simulink model "simscape_Example_20231128_1528"  (R2023b)
settings: Solver=ode23t  StartTime=0.0  StopTime=100  RelTol=1e-3
libraries: nesl_utility x8, fl_lib x6, ee_lib x4
settings Model: Creator=Patri  LastModifiedBy=Patri

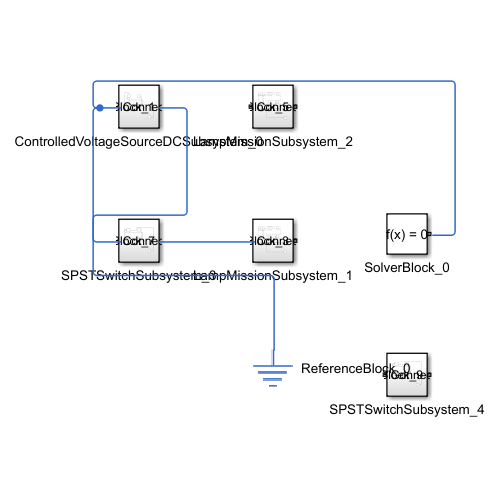
[thumbnail: Simulink's stored preview of the top-level diagram]
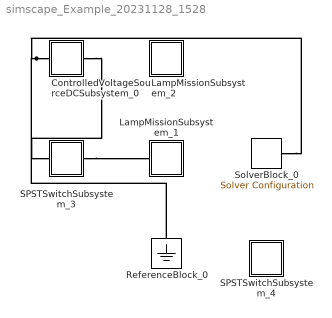
== system simscape_Example_20231128_1528 ==
  ControlledVoltageSourceDCSubsystem_0 : Subsystem
  LampMissionSubsystem_1 : Subsystem
  LampMissionSubsystem_2 : Subsystem
  ReferenceBlock_0 : fl_lib/Electrical/Electrical Elements/Electrical Reference
  SPSTSwitchSubsystem_3 : Subsystem
  SPSTSwitchSubsystem_4 : Subsystem
  SolverBlock_0 : nesl_utility/Solver Configuration  PhysicalDomain=network_engine_domain  SubClassName=solver  LeftPortType=input  RightPortType=generic  Tones=[]  Harmonics=[]  SimulateNoise=off  Profile=off  UseLocalSampling=off  EnableSwitchedLinearOptims=on  FrequencyDomain=off  UseCCode=off  RelTol=0.001  AbsTol=0.001  MinStep=1e-09  ToWorkspace=off  RevertToSquareIcSolve=off  NumHomotopyIterations=100  PhasorMode=off  PhasorModeNumHarmonics=1  ConsistencySolver=NEWTON_XTOL_AFTER_FTOL  IndexReductionMethod=DerivativeReplacement  DoDC=off  ResidualTolerance=1e-09  ConsistencyTolSource=GLOBAL  ConsistencyAbsTol=0.001  ConsistencyRelTol=0.001  ConsistencyTolFactor=0.001  UseLocalSolver=off  LocalSolverChoice=NE_BACKWARD_EULER_ADVANCER  ResolveIndetEquations=on  FunctionEvalNumThread=1  LocalSolverSampleTime=0.001  DoFixedCost=off  MaxNonlinIter=3  MaxModeIter=2  ComputeImpulses=off  ImpulseIterations=2  LinearAlgebra=auto  LinearAlgebraNumThread=0  EquationFormulation=NE_TIME_EF  DelaysMemoryBudget=1024  AutomaticFiltering=on  FilteringTimeConstant=0.001  PartitionStorageMethod=AS_NEEDED  PartitionMemoryBudget=1024  PartitionMethod=ROBUST  MultibodyUseLocalSolver=off  MultibodyLocalSolverChoice=ODE1  MultibodyLocalSolverSampleTime=0.001
  connections:
  ControlledVoltageSourceDCSubsystem_0/RConn1 -- SPSTSwitchSubsystem_3/LConn1
  SPSTSwitchSubsystem_3/RConn1 -- LampMissionSubsystem_1/LConn1
  ControlledVoltageSourceDCSubsystem_0/LConn1 -- SolverBlock_0/RConn1 -- ReferenceBlock_0/LConn1

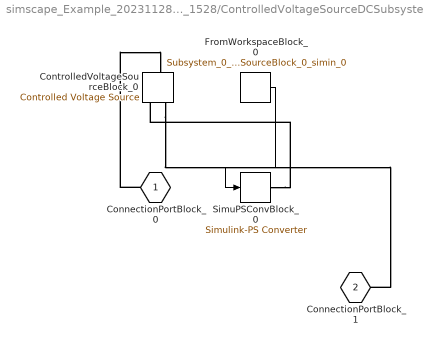
== system simscape_Example_20231128_1528/ControlledVoltageSourceDCSubsystem_0 ==
  ControlledVoltageSourceBlock_0 : fl_lib/Electrical/Electrical Sources/Controlled Voltage Source
  FromWorkspaceBlock_0 : FromWorkspace  VariableName=Subsystem_0_ControlledVoltageSourceBlock_0_simin_0
  SimuPSConvBlock_0 : nesl_utility/Simulink-PS Converter  PhysicalDomain=network_engine_domain  SubClassName=ps_input  LeftPortType=input  RightPortType=output  PseudoPeriodic=off  Frequencies=[]  NoiseDistribution=none  NoiseParameters=[]  Unit=1  AffineConversion=off  FilteringAndDerivatives=filter  SimscapeFilterOrder=1  InputFilterTimeConstant=0.001  UdotUserProvided=0
  ConnectionPortBlock_0 : PMIOPort  Side=Left
  ConnectionPortBlock_1 : PMIOPort  Port=2  Side=Right
  wires:
  FromWorkspaceBlock_0/1 -> SimuPSConvBlock_0/1
  connections:
  SimuPSConvBlock_0/RConn1 -- ControlledVoltageSourceBlock_0/RConn1
  ConnectionPortBlock_0/RConn1 -- ControlledVoltageSourceBlock_0/LConn1
  ControlledVoltageSourceBlock_0/RConn2 -- ConnectionPortBlock_1/RConn1

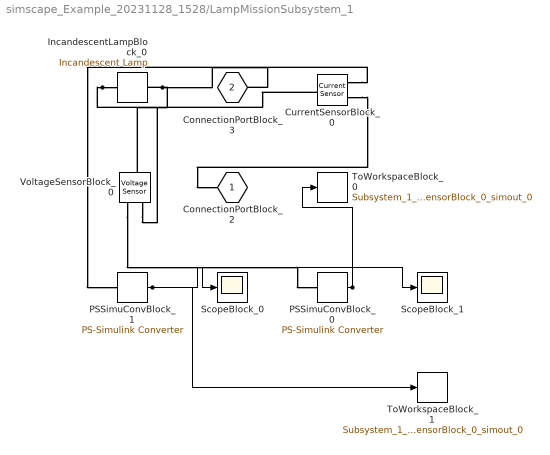
== system simscape_Example_20231128_1528/LampMissionSubsystem_1 ==
  CurrentSensorBlock_0 : fl_lib/Electrical/Electrical Sensors/Current Sensor
  IncandescentLampBlock_0 : ee_lib/Passive/Incandescent Lamp  R_param=ee.enum.passive.lampParam.specifyR  R0=0.15 Ohm  R1=1.0 Ohm  i0=70 A  i1=10 A  Vrated=12.0 V  alpha=0.004 1/K  tc=25 ms  initial_state=simscape.enum.onoff.off  enable_fault=simscape.enum.onoff.off  t_fault=inf s  R_fault=1e6 Ohm
      settings: InternalSimscapePortConfiguration="{\"Bottom\":[],\"Left\":[{\"id\":\"p\",\"label\":\"+\",\"type\":\"foundation.electrical.electrical\"}],\"Right\":[{\"id\":\"n\",\"label\":\"-\",\"type\":\"foundation.electrical.electrical\"}],\"Top\":[]}"
  PSSimuConvBlock_0 : nesl_utility/PS-Simulink Converter  PhysicalDomain=network_engine_domain  SubClassName=ps_output  LeftPortType=input  RightPortType=output  PseudoPeriodic=off  Frequencies=[]  VectorFormat=inherit  Unit=inherit  AffineConversion=off
  PSSimuConvBlock_1 : nesl_utility/PS-Simulink Converter  PhysicalDomain=network_engine_domain  SubClassName=ps_output  LeftPortType=input  RightPortType=output  PseudoPeriodic=off  Frequencies=[]  VectorFormat=inherit  Unit=inherit  AffineConversion=off
  ScopeBlock_0 : Scope
  ScopeBlock_1 : Scope
  ToWorkspaceBlock_0 : ToWorkspace  VariableName=Subsystem_1_VoltageSensorBlock_0_simout_0  SaveFormat=Structure With Time
  ToWorkspaceBlock_1 : ToWorkspace  VariableName=Subsystem_1_CurrentSensorBlock_0_simout_0  SaveFormat=Structure With Time
  VoltageSensorBlock_0 : fl_lib/Electrical/Electrical Sensors/Voltage Sensor
  ConnectionPortBlock_2 : PMIOPort  Side=Left
  ConnectionPortBlock_3 : PMIOPort  Port=2  Side=Right
  wires:
  PSSimuConvBlock_0/1 -> ToWorkspaceBlock_0/1, ScopeBlock_0/1
  PSSimuConvBlock_1/1 -> ToWorkspaceBlock_1/1, ScopeBlock_1/1
  connections:
  VoltageSensorBlock_0/RConn1 -- PSSimuConvBlock_0/LConn1
  IncandescentLampBlock_0/LConn1 -- VoltageSensorBlock_0/RConn2 -- CurrentSensorBlock_0/LConn1
  IncandescentLampBlock_0/RConn1 -- VoltageSensorBlock_0/LConn1 -- ConnectionPortBlock_3/RConn1
  CurrentSensorBlock_0/RConn1 -- PSSimuConvBlock_1/LConn1
  CurrentSensorBlock_0/RConn2 -- ConnectionPortBlock_2/RConn1

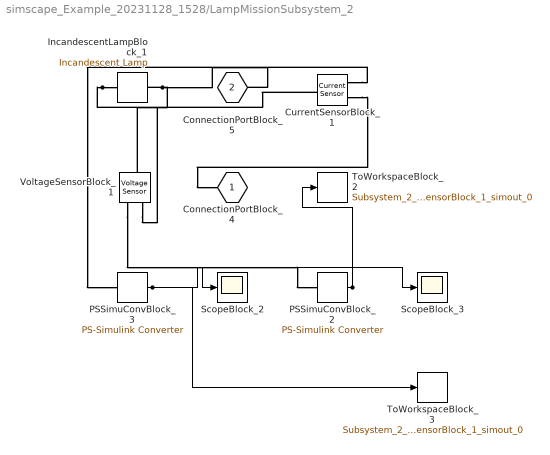
== system simscape_Example_20231128_1528/LampMissionSubsystem_2 ==
  CurrentSensorBlock_1 : fl_lib/Electrical/Electrical Sensors/Current Sensor
  IncandescentLampBlock_1 : ee_lib/Passive/Incandescent Lamp  R_param=ee.enum.passive.lampParam.specifyR  R0=0.15 Ohm  R1=1.0 Ohm  i0=70 A  i1=10 A  Vrated=12.0 V  alpha=0.004 1/K  tc=25 ms  initial_state=simscape.enum.onoff.off  enable_fault=simscape.enum.onoff.off  t_fault=inf s  R_fault=1e6 Ohm
      settings: InternalSimscapePortConfiguration="{\"Bottom\":[],\"Left\":[{\"id\":\"p\",\"label\":\"+\",\"type\":\"foundation.electrical.electrical\"}],\"Right\":[{\"id\":\"n\",\"label\":\"-\",\"type\":\"foundation.electrical.electrical\"}],\"Top\":[]}"
  PSSimuConvBlock_2 : nesl_utility/PS-Simulink Converter  PhysicalDomain=network_engine_domain  SubClassName=ps_output  LeftPortType=input  RightPortType=output  PseudoPeriodic=off  Frequencies=[]  VectorFormat=inherit  Unit=inherit  AffineConversion=off
  PSSimuConvBlock_3 : nesl_utility/PS-Simulink Converter  PhysicalDomain=network_engine_domain  SubClassName=ps_output  LeftPortType=input  RightPortType=output  PseudoPeriodic=off  Frequencies=[]  VectorFormat=inherit  Unit=inherit  AffineConversion=off
  ScopeBlock_2 : Scope
  ScopeBlock_3 : Scope
  ToWorkspaceBlock_2 : ToWorkspace  VariableName=Subsystem_2_VoltageSensorBlock_1_simout_0  SaveFormat=Structure With Time
  ToWorkspaceBlock_3 : ToWorkspace  VariableName=Subsystem_2_CurrentSensorBlock_1_simout_0  SaveFormat=Structure With Time
  VoltageSensorBlock_1 : fl_lib/Electrical/Electrical Sensors/Voltage Sensor
  ConnectionPortBlock_4 : PMIOPort  Side=Left
  ConnectionPortBlock_5 : PMIOPort  Port=2  Side=Right
  wires:
  PSSimuConvBlock_2/1 -> ToWorkspaceBlock_2/1, ScopeBlock_2/1
  PSSimuConvBlock_3/1 -> ToWorkspaceBlock_3/1, ScopeBlock_3/1
  connections:
  VoltageSensorBlock_1/RConn1 -- PSSimuConvBlock_2/LConn1
  IncandescentLampBlock_1/LConn1 -- VoltageSensorBlock_1/RConn2 -- CurrentSensorBlock_1/LConn1
  IncandescentLampBlock_1/RConn1 -- VoltageSensorBlock_1/LConn1 -- ConnectionPortBlock_5/RConn1
  CurrentSensorBlock_1/RConn1 -- PSSimuConvBlock_3/LConn1
  CurrentSensorBlock_1/RConn2 -- ConnectionPortBlock_4/RConn1

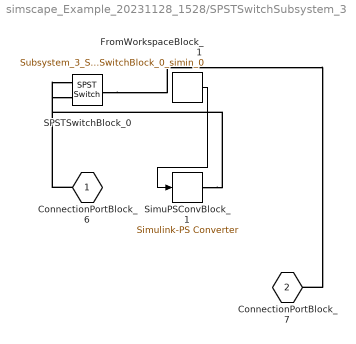
== system simscape_Example_20231128_1528/SPSTSwitchSubsystem_3 ==
  FromWorkspaceBlock_1 : FromWorkspace  VariableName=Subsystem_3_SPSTSwitchBlock_0_simin_0
  SPSTSwitchBlock_0 : ee_lib/Switches & Breakers/SPST Switch  R_closed=0.01 Ohm  G_open=1e-6 S  Threshold=0.5 V  Width=0 V  model_dynamics=0  t_on=1e-3 s  t_off=1e-3 s  initial_vT=0 V
      settings: InternalSimscapePortConfiguration="{\"Bottom\":[],\"Left\":[{\"id\":\"vT\",\"label\":\"vT\",\"type\":\"input\"},{\"id\":\"p\",\"label\":\"\",\"type\":\"foundation.electrical.electrical\"}],\"Right\":[{\"id\":\"n\",\"label\":\"\",\"type\":\"foundation.electrical.electrical\"}],\"Top\":[]}"
  SimuPSConvBlock_1 : nesl_utility/Simulink-PS Converter  PhysicalDomain=network_engine_domain  SubClassName=ps_input  LeftPortType=input  RightPortType=output  PseudoPeriodic=off  Frequencies=[]  NoiseDistribution=none  NoiseParameters=[]  Unit=1  AffineConversion=off  FilteringAndDerivatives=filter  SimscapeFilterOrder=1  InputFilterTimeConstant=0.001  UdotUserProvided=0
  ConnectionPortBlock_6 : PMIOPort  Side=Left
  ConnectionPortBlock_7 : PMIOPort  Port=2  Side=Right
  wires:
  FromWorkspaceBlock_1/1 -> SimuPSConvBlock_1/1
  connections:
  SimuPSConvBlock_1/RConn1 -- SPSTSwitchBlock_0/LConn1
  ConnectionPortBlock_6/RConn1 -- SPSTSwitchBlock_0/LConn2
  SPSTSwitchBlock_0/RConn1 -- ConnectionPortBlock_7/RConn1

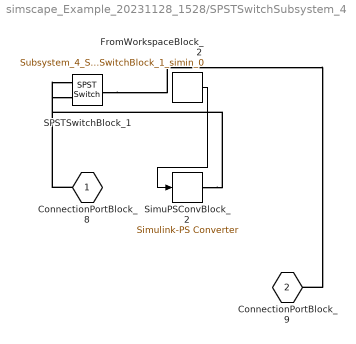
== system simscape_Example_20231128_1528/SPSTSwitchSubsystem_4 ==
  FromWorkspaceBlock_2 : FromWorkspace  VariableName=Subsystem_4_SPSTSwitchBlock_1_simin_0
  SPSTSwitchBlock_1 : ee_lib/Switches & Breakers/SPST Switch  R_closed=0.01 Ohm  G_open=1e-6 S  Threshold=0.5 V  Width=0 V  model_dynamics=0  t_on=1e-3 s  t_off=1e-3 s  initial_vT=0 V
      settings: InternalSimscapePortConfiguration="{\"Bottom\":[],\"Left\":[{\"id\":\"vT\",\"label\":\"vT\",\"type\":\"input\"},{\"id\":\"p\",\"label\":\"\",\"type\":\"foundation.electrical.electrical\"}],\"Right\":[{\"id\":\"n\",\"label\":\"\",\"type\":\"foundation.electrical.electrical\"}],\"Top\":[]}"
  SimuPSConvBlock_2 : nesl_utility/Simulink-PS Converter  PhysicalDomain=network_engine_domain  SubClassName=ps_input  LeftPortType=input  RightPortType=output  PseudoPeriodic=off  Frequencies=[]  NoiseDistribution=none  NoiseParameters=[]  Unit=1  AffineConversion=off  FilteringAndDerivatives=filter  SimscapeFilterOrder=1  InputFilterTimeConstant=0.001  UdotUserProvided=0
  ConnectionPortBlock_8 : PMIOPort  Side=Left
  ConnectionPortBlock_9 : PMIOPort  Port=2  Side=Right
  wires:
  FromWorkspaceBlock_2/1 -> SimuPSConvBlock_2/1
  connections:
  SimuPSConvBlock_2/RConn1 -- SPSTSwitchBlock_1/LConn1
  ConnectionPortBlock_8/RConn1 -- SPSTSwitchBlock_1/LConn2
  SPSTSwitchBlock_1/RConn1 -- ConnectionPortBlock_9/RConn1
